simulink model "e5_taller_se"  (R2018a)
settings: Solver=VariableStepAuto  StartTime=0.0  StopTime=0.9  RelTol=1e-3
InitFcn:
  | ejercicio_5_taller_se
values from neighbouring files (symbols this model uses):
  A = [-1/(R*C) -1/C;1/L 0]    [ejemplo_se.m]    (also in ejercicio_5_taller_se.m = [0 -1/L 0; 1/C1 -1/(R*C1) 1/(R*C1); 0 1/(R*C2) -1/(R*C2)])
  B = [1/C 0]'    [ejemplo_se.m]    (also in ejercicio_5_taller_se.m = [1/L 0 0]')
  C = 12e-6    (= 1.2e-05)    [ejemplo_se.m]    (also in ejercicio_5_taller_se.m = [0 0 1])
  C1 = 1e-6    (= 1e-06)    [ejercicio_5_taller_se.m]
  C2 = 10e-6    (= 1e-05)    [ejercicio_5_taller_se.m]
  h = tf([R*L 0],[R*C*L L R])    [ejemplo_se.m]    (also in ejercicio_5_taller_se.m = tf(1,[L*R*C1*C2 L*(C1+C2) R*C2 1]); po.m = tf(k,[tao 1]))
  L = 100e-3    (= 0.1)    [ejemplo_se.m]    (also in ejercicio_5_taller_se.m = 0.5)
  R = 1e3    (= 1000)    [ejemplo_se.m]    (also in ejercicio_5_taller_se.m = 10000)
settings Model: Creator=carma  LastModifiedBy=carma

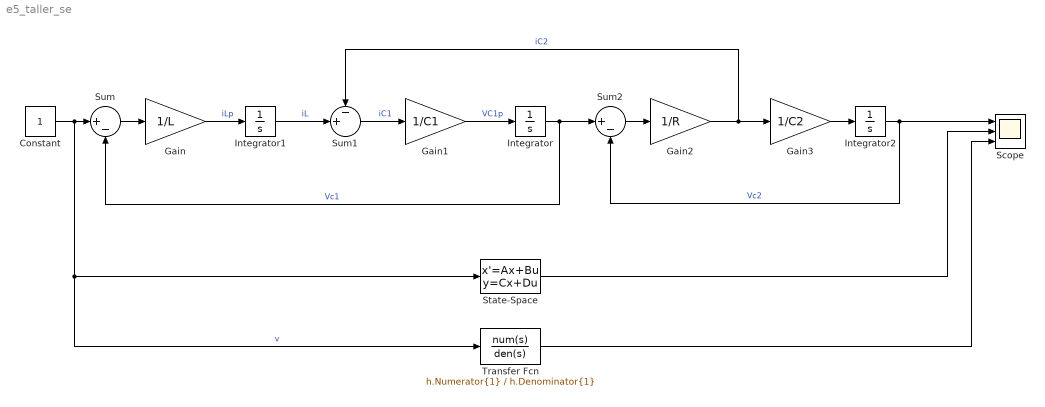
== system e5_taller_se ==
  Constant : Constant
  Gain : Gain  Gain=1/L
  Gain1 : Gain  Gain=1/C1
  Gain2 : Gain  Gain=1/R
  Gain3 : Gain  Gain=1/C2
  Integrator : Integrator
  Integrator1 : Integrator
  Integrator2 : Integrator
  Scope : Scope  NumInputPorts=3
  State-Space : StateSpace  A=A  B=B  C=C  D=0  InitialCondition=0
  Sum : Sum  Inputs=|+-
  Sum1 : Sum  Inputs=-+|
  Sum2 : Sum  Inputs=|+-
  Transfer Fcn : TransferFcn  Numerator=h.Numerator{1}  Denominator=h.Denominator{1}
  wires:
  Sum/1 -> Gain/1
  Constant/1 -> Transfer Fcn/1, State-Space/1, Sum/1  "v"
  Integrator/1 -> Sum2/1, Sum/2  "Vc1"
  Gain/1 -> Integrator1/1  "iLp"
  Sum1/1 -> Gain1/1  "iC1"
  Integrator1/1 -> Sum1/2  "iL"
  Gain1/1 -> Integrator/1  "VC1p"
  Gain2/1 -> Sum1/1, Gain3/1  "iC2"
  Sum2/1 -> Gain2/1
  Gain3/1 -> Integrator2/1
  Integrator2/1 -> Scope/1, Sum2/2  "Vc2"
  State-Space/1 -> Scope/2
  Transfer Fcn/1 -> Scope/3
